simulink model "Task9ss"  (R2017b)
settings: Solver=VariableStepAuto  StartTime=0.0  StopTime=10  RelTol=1e-3
values from neighbouring files (symbols this model uses):
  A1 = Ask    [H_inf_ctrl.m]    (also in Task8.m = [0 1 0 0;-(k1+k2)/m 0 (l1*k1-l2*k2)/m 0; 0 0 0 1;-(l1*k1-l2*)
  B1 = Bsk    [H_inf_ctrl.m]    (also in Task8.m = [0 0 0 0;k1/m k2/m 1/m 1/m;0 0 0 0;-k1*l1/J k2*l2/J -l1/J l2)
  C1 = Csk    [H_inf_ctrl.m]    (also in Task8.m = eye(4))
  c_x = cx(i)    [Task8.m]
  c_z = 190000    [Task8.m]
  D1 = Dsk    [H_inf_ctrl.m]    (also in Task8.m = zeros(4))
  f = 8    [H_inf_ctrl.m]    (also in Task6.m = 2; Task8.m; task5.m = 0.5)
  l1 = L    (= 6)    [H_inf_ctrl.m]    (also in Task8.m)
  l2 = L    (= 6)    [H_inf_ctrl.m]    (also in Task8.m)
  src = 1    [H_inf_ctrl.m]    (also in Task3.m = 3; Task6.m = 3; Task8.m)
undefined symbols (not defined in the file or in its folder): sigbuilder_block
settings Model: Creator=Dell  LastModifiedBy=Dell

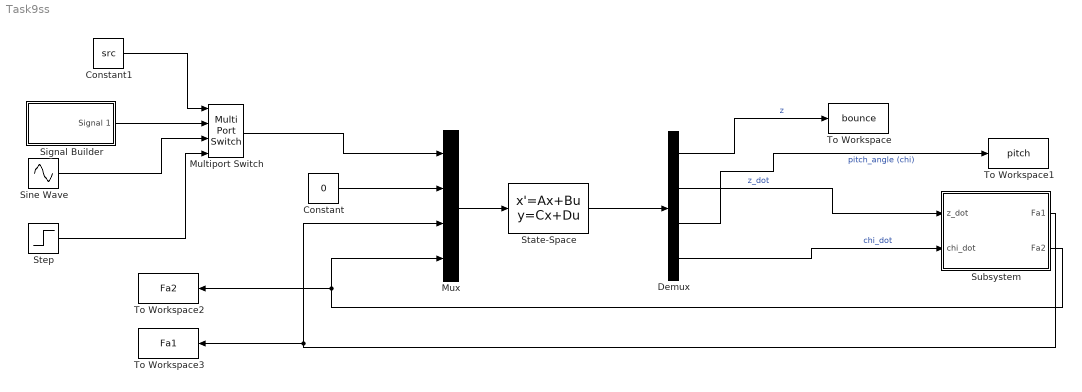
== system Task9ss ==
  Constant : Constant  Value=0
  Constant1 : Constant  Value=src
  Demux : Demux
  Multiport Switch : MultiPortSwitch
  Mux : Mux
  Signal Builder : Subsystem  Tag=STV Subsys  LoadFcn=sigbuilder_block('load');  StartFcn=sigbuilder_block('start');  StopFcn=sigbuilder_block('stop');  ClipboardFcn=sigbuilder_block('clipboard');  mask(Sigbuilder block){tuvar=[0:10]}
      mask help: Simulink:masks:SigbuilderBlock_MD
      mask init:
      | if ~strcmp(get_param(bdroot(gcbh),'SimulationStatus'),'stopped') tuvar = sigbuilder_block('maskInit'); end
      settings: CopyFcn=sigbuilder_block('copy');  DeleteFcn=sigbuilder_block('delete');  ModelCloseFcn=sigbuilder_block('modelClose');  PreSaveFcn=sigbuilder_block('preSave');  PauseFcn=sigbuilder_block('pause');  ContinueFcn=sigbuilder_block('continue');  NameChangeFcn=sigbuilder_block('namechange');  OpenFcn=sigbuilder_block('open',[437.6 199.2 550.4 400 ]);  CloseFcn=sigbuilder_block('close');
      mask Display: plot(0, 0, 100, 100,[2, 2, 32, 32, 2], [68, 8, 8, 68, 68],[32, 2], [38, 38], [32, 19, 2],[53, 60, 44], [32, 17, 17, 2],[16, 16, 31, 31]);txt = getActiveGroup(gcbh);text(2, 100, txt,'verticalAlignment', 'top');
  Sine Wave : Sin  Amplitude=0.01  Frequency=2*pi*f  SampleTime=0
  State-Space : StateSpace  A=A1  B=B1  C=C1  D=D1  InitialCondition=0
  Step : Step  SampleTime=0
  Subsystem : Subsystem
  To Workspace : ToWorkspace  VariableName=bounce  SaveFormat=Timeseries  SampleTime=-1
  To Workspace1 : ToWorkspace  VariableName=pitch  SaveFormat=Timeseries  SampleTime=-1
  To Workspace2 : ToWorkspace  VariableName=Fa2  SaveFormat=Timeseries  SampleTime=-1
  To Workspace3 : ToWorkspace  VariableName=Fa1  SaveFormat=Timeseries  SampleTime=-1
  wires:
  Constant/1 -> Mux/2
  State-Space/1 -> Demux/1
  Multiport Switch/1 -> Mux/1
  Constant1/1 -> Multiport Switch/1
  Sine Wave/1 -> Multiport Switch/3
  Signal Builder/1(Signal 1) -> Multiport Switch/2
  Mux/1 -> State-Space/1
  Demux/1 -> To Workspace/1  "z"
  Demux/3 -> To Workspace1/1  "pitch_angle (chi)"
  Step/1 -> Multiport Switch/4
  Demux/2 -> Subsystem/1(z_dot)  "z_dot"
  Demux/4 -> Subsystem/2(chi_dot)  "chi_dot"
  Subsystem/1(Fa1) -> To Workspace3/1, Mux/3
  Subsystem/2(Fa2) -> To Workspace2/1, Mux/4

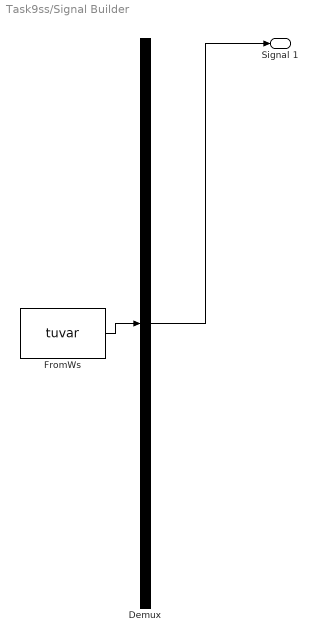
== system Task9ss/Signal Builder ==
  Demux : Demux  Tag=STV Demux  Outputs=1
  FromWs : FromWorkspace  Tag=STV FromWs  VariableName=tuvar  SampleTime=0
      SigBuilderData=|
      | common.afterFinalStr = 'Extrapolate'
      | common.sampleTime = 0
      | dataSet.timeRange = [0 10]
      | dataSet.name = 'Group 1'
      | sbobj.Groups.Name = 'Group 1'
      | sbobj.Groups.Signals.Name = 'Signal 1'
      | sbobj.Groups.Signals.XData = [0 1 1 4.62 10]
      | sbobj.Groups.Signals.YData = [0.03 0.03 0 0 0]
  Signal 1 : Outport  Tag=STV Outport
  wires:
  Demux/1 -> Signal 1/1
  FromWs/1 -> Demux/1

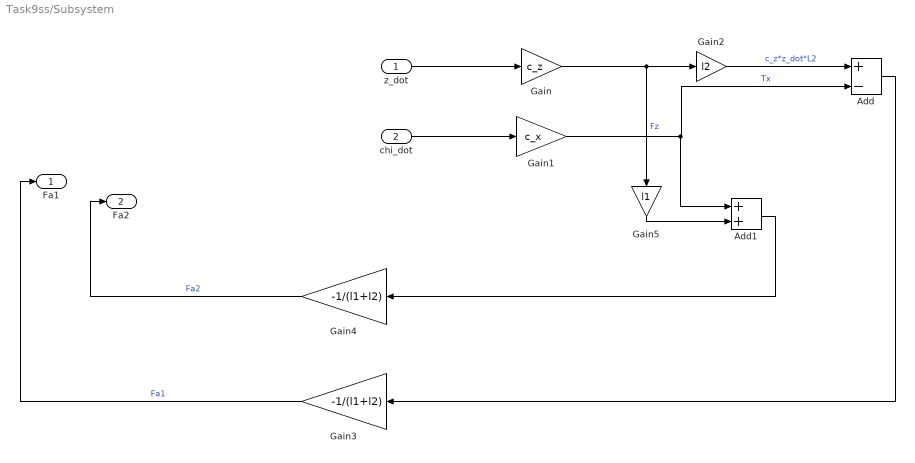
== system Task9ss/Subsystem ==
  z_dot : Inport
  chi_dot : Inport  Port=2
  Add : Sum  Inputs=+-
  Add1 : Sum
  Gain : Gain  Gain=c_z
  Gain1 : Gain  Gain=c_x
  Gain2 : Gain  Gain=l2
  Gain3 : Gain  Gain=-1/(l1+l2)
  Gain4 : Gain  Gain=-1/(l1+l2)
  Gain5 : Gain  Gain=l1
  Fa1 : Outport
  Fa2 : Outport  Port=2
  wires:
  Gain2/1 -> Add/1  "c_z*z_dot*L2"
  z_dot/1 -> Gain/1
  Gain1/1 -> Add1/1, Add/2  "Tx"
  chi_dot/1 -> Gain1/1
  Gain3/1 -> Fa1/1  "Fa1"
  Add/1 -> Gain3/1
  Gain4/1 -> Fa2/1  "Fa2"
  Add1/1 -> Gain4/1
  Gain/1 -> Gain5/1, Gain2/1  "Fz"
  Gain5/1 -> Add1/2
